simulink model "circuito_Motor_DC"  (R2019a)
settings: Solver=VariableStepAuto  StartTime=0.0  StopTime=10.0  RelTol=1e-3
values from neighbouring files (symbols this model uses):
  Ke = 0.4    [motorDC_matlab.m]
  Kf = 0.001    [motorDC_matlab.m]
  La = 10e-3    (= 0.01)    [motorDC_matlab.m]
  Ra = 0.5    [motorDC_matlab.m]
settings Model: Creator=User  LastModifiedBy=User
settings DebuggingCC: ArithmeticOperatorsInVariantConditions=warning

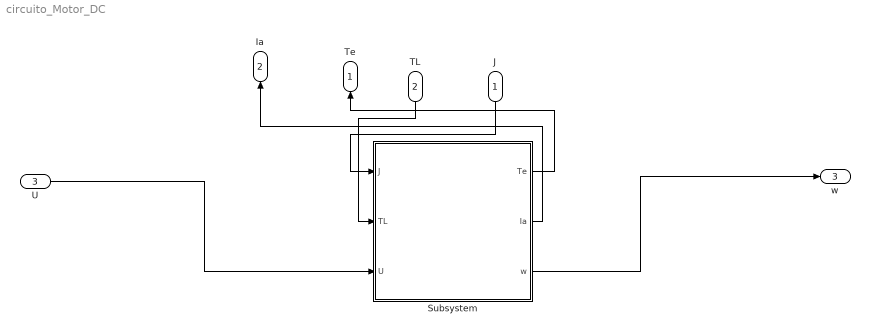
== system circuito_Motor_DC ==
  J : Inport
  TL : Inport  Port=2
  U : Inport  Port=3
  Subsystem : Subsystem
  Te : Outport
  Ia : Outport  Port=2
  w : Outport  Port=3
  wires:
  J/1 -> Subsystem/1(J)
  TL/1 -> Subsystem/2(TL)
  U/1 -> Subsystem/3(U)
  Subsystem/1(Te) -> Te/1
  Subsystem/2(Ia) -> Ia/1
  Subsystem/3(w) -> w/1

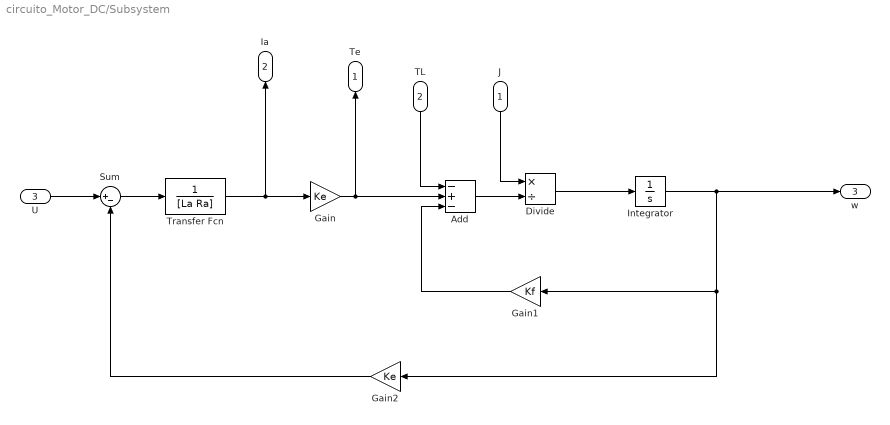
== system circuito_Motor_DC/Subsystem ==
  J : Inport
  TL : Inport  Port=2
  U : Inport  Port=3
  Add : Sum  Inputs=-+-
  Divide : Product  Inputs=*/
  Gain : Gain  Gain=Ke
  Gain1 : Gain  Gain=Kf
  Gain2 : Gain  Gain=Ke
  Integrator : Integrator
  Sum : Sum  Inputs=|+-
  Transfer Fcn : TransferFcn  Denominator=[La Ra]
  Te : Outport
  Ia : Outport  Port=2
  w : Outport  Port=3
  wires:
  Sum/1 -> Transfer Fcn/1
  Add/1 -> Divide/2
  J/1 -> Divide/1
  Integrator/1 -> w/1, Gain2/1, Gain1/1
  Transfer Fcn/1 -> Ia/1, Gain/1
  U/1 -> Sum/1
  Gain2/1 -> Sum/2
  Gain/1 -> Te/1, Add/2
  Gain1/1 -> Add/3
  TL/1 -> Add/1
  Divide/1 -> Integrator/1
